simulink library "INT_Prp_TrqDesCoord"  (R2016b)
settings: Solver=VariableStepAuto  StartTime=0.0  StopTime=10.0  RelTol=1e-3
settings Model: Creator=Administrator  LastModifiedBy=Administrator

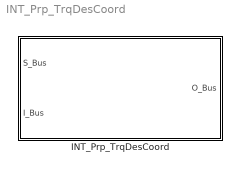
== system INT_Prp_TrqDesCoord ==
  INT_Prp_TrqDesCoord : Subsystem

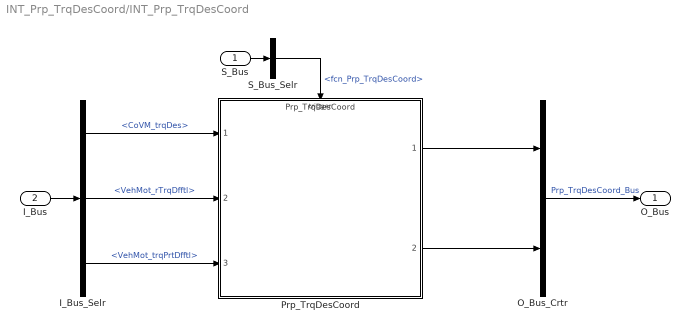
== system INT_Prp_TrqDesCoord/INT_Prp_TrqDesCoord ==
  S_Bus : Inport
  I_Bus : Inport  Port=2
  I_Bus_Selr : BusSelector  OutputSignals=CoVM_trqDes,VehMot_rTrqDfftl,VehMot_trqPrtDfftl
  O_Bus_Crtr : BusCreator  Inputs=2
  Prp_TrqDesCoord : ModelReference  ModelNameDialog=Prp_TrqDesCoord  SimulationMode=Normal  ModelReferenceVersion=1.2  TriggerPortName=function  TriggerPortTriggerType=function-call  TriggerPortStatesWhenEnabling=held
  S_Bus_Selr : BusSelector  OutputSignals=fcn_Prp_TrqDesCoord
  O_Bus : Outport
  wires:
  S_Bus_Selr/1 -> Prp_TrqDesCoord/Trigger  "<fcn_Prp_TrqDesCoord>"
  S_Bus/1 -> S_Bus_Selr/1
  I_Bus/1 -> I_Bus_Selr/1
  I_Bus_Selr/1 -> Prp_TrqDesCoord/1  "<CoVM_trqDes>"
  I_Bus_Selr/2 -> Prp_TrqDesCoord/2  "<VehMot_rTrqDfftl>"
  I_Bus_Selr/3 -> Prp_TrqDesCoord/3  "<VehMot_trqPrtDfftl>"
  O_Bus_Crtr/1 -> O_Bus/1  "Prp_TrqDesCoord_Bus"
  Prp_TrqDesCoord/1 -> O_Bus_Crtr/1
  Prp_TrqDesCoord/2 -> O_Bus_Crtr/2
